simulink model "APP_VD"  (R2016b)
settings: configuration reference "CodeGenConfigSet" (kept outside this file)
values from neighbouring files (symbols this model uses):
  APP_drLinRmp_C = Calibration.Parameter    [init_APP_VD.m]
  APP_facLowNegPT1_C = Calibration.Parameter    [init_APP_VD.m]
  APP_facLowPosPT1_C = Calibration.Parameter    [init_APP_VD.m]
  APP_facMidNegPT1_C = Calibration.Parameter    [init_APP_VD.m]
  APP_facMidPosPT1_C = Calibration.Parameter    [init_APP_VD.m]
  APP_facUppNegPT1_C = Calibration.Parameter    [init_APP_VD.m]
  APP_facUppPosPT1_C = Calibration.Parameter    [init_APP_VD.m]
  APP_rThrFltLowNeg_C = Calibration.Parameter    [init_APP_VD.m]
  APP_rThrFltLowPos_C = Calibration.Parameter    [init_APP_VD.m]
  APP_rThrFltMidNeg_C = Calibration.Parameter    [init_APP_VD.m]
  APP_rThrFltMidPos_C = Calibration.Parameter    [init_APP_VD.m]
  APP_swtEnaFlt_C = Calibration.Parameter    [init_APP_VD.m]
  APP_swtEnaUnJit_C = Calibration.Parameter    [init_APP_VD.m]
  APP_uJitter_C = Calibration.Parameter    [init_APP_VD.m]
  MoFAPP_rLinAPPCURCalMsgA_CUR = Calibration.Parameter    [init_APP_VD.m]
  MoFAPP_rLinAPPCURCalMsgA_CURX = Calibration.Parameter    [init_APP_VD.m]
  SigTst_rAPP_C = Calibration.Parameter    [init_APP_VD.m]
  SigTst_swtAPP_C = Calibration.Parameter    [init_APP_VD.m]
undefined symbols (not defined in the file or in its folder): APP_VD_DT, Switch_conv
libraries: CXLib x4
settings Model: Creator=lenovo  LastModifiedBy=zhoutinglin
settings ConfigSetRef: SourceLocation=Base Workspace

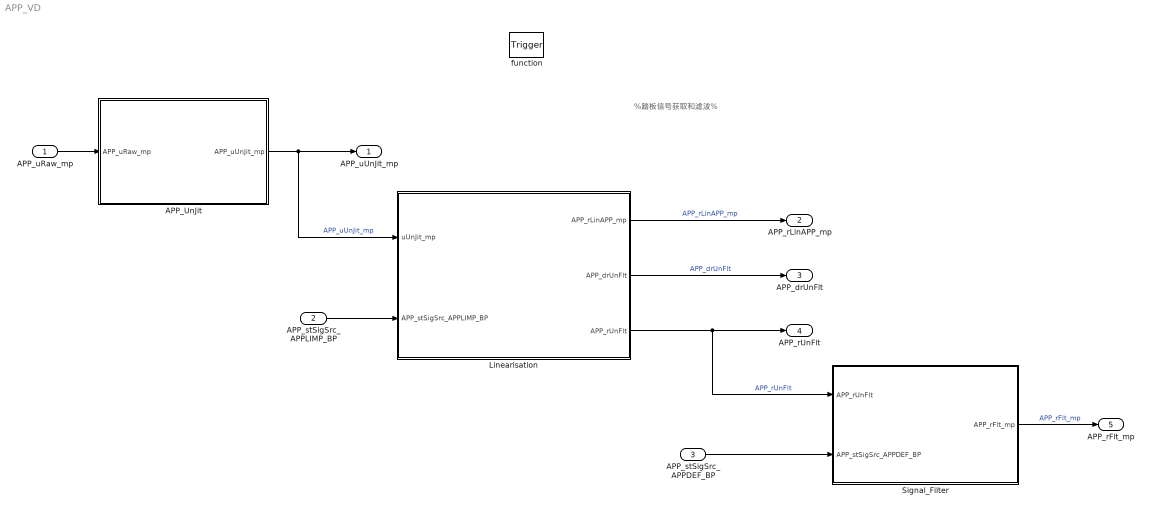
== system APP_VD ==
  note: %踏板信号获取和滤波%
  APP_uRaw_mp : Inport  Tag=mv  Description=Acceleration pedal position raw value  OutMin=0  OutMax=5000  OutDataTypeStr=Ad_mv
  APP_stSigSrc_APPLIMP_BP : Inport  Description=Substitute operation active, accelerator pedal sensor value and accelerator pedal sensor increase are limited  Port=2  OutMin=0  OutMax=1  OutDataTypeStr=boolean
  APP_stSigSrc_APPDEF_BP : Inport  Description=both the sensors are defective. Use the default value  Port=3  OutMin=0  OutMax=1  OutDataTypeStr=boolean
  function : TriggerPort  TriggerType=function-call  VariantControl=Variant
  APP_UnJit : Subsystem
  Linearisation : Subsystem
  Signal_Filter : Subsystem
  APP_uUnJit_mp : Outport  Tag=mv  Description=Acceleration pedal position unjittered value  OutMin=0  OutMax=5000  OutDataTypeStr=Ad_mv
  APP_rLinAPP_mp : Outport  Tag=%  Description=Linearisation ratio of accelerator pedal  Port=2  OutMin=0  OutMax=100  OutDataTypeStr=Accpedal_rate
  APP_drUnFlt : Outport  Tag=%/s  Description=Acceleration pedal position gradient of unfilterd value  Port=3  OutMin=-100000  OutMax=100000  OutDataTypeStr=Accpedal_rate_s
  APP_rUnFlt : Outport  Tag=%  Description=Unfiltered APP value  Port=4  OutMin=0  OutMax=100  OutDataTypeStr=Accpedal_rate
  APP_rFlt_mp : Outport  Tag=%  Description=Acceleration pedal position filtered value  Port=5  OutMin=0  OutMax=100  OutDataTypeStr=Accpedal_rate
  wires:
  APP_uRaw_mp/1 -> APP_UnJit/1(APP_uRaw_mp)
  Linearisation/3(APP_rUnFlt) -> APP_rUnFlt/1, Signal_Filter/1(APP_rUnFlt)  "APP_rUnFlt"
  APP_UnJit/1(APP_uUnJit_mp) -> APP_uUnJit_mp/1, Linearisation/1(uUnJit_mp)  "APP_uUnJit_mp"
  APP_stSigSrc_APPLIMP_BP/1 -> Linearisation/2(APP_stSigSrc_APPLIMP_BP)
  Linearisation/1(APP_rLinAPP_mp) -> APP_rLinAPP_mp/1  "APP_rLinAPP_mp"
  Linearisation/2(APP_drUnFlt) -> APP_drUnFlt/1  "APP_drUnFlt"
  APP_stSigSrc_APPDEF_BP/1 -> Signal_Filter/2(APP_stSigSrc_APPDEF_BP)
  Signal_Filter/1(APP_rFlt_mp) -> APP_rFlt_mp/1  "APP_rFlt_mp"

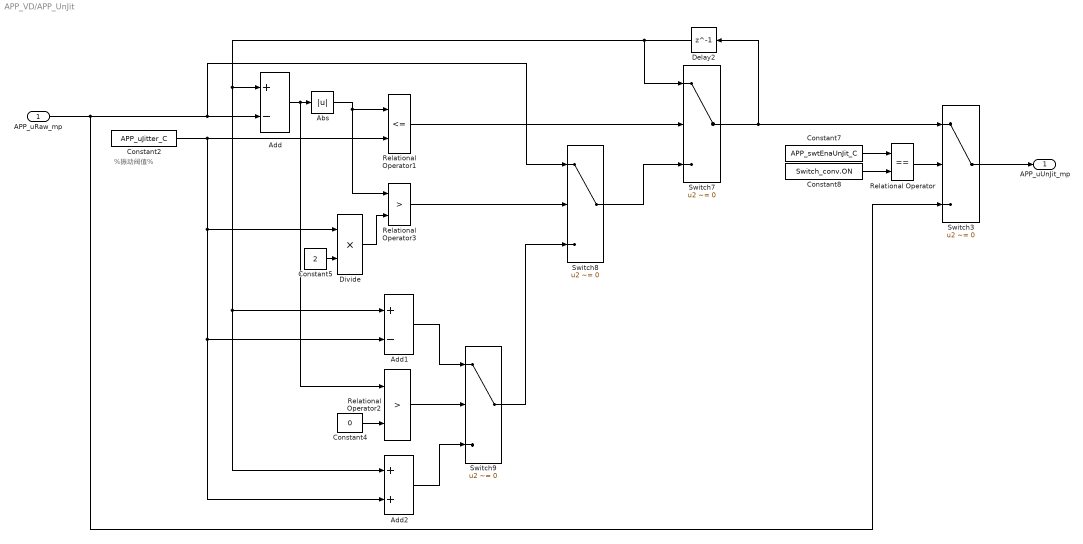
== system APP_VD/APP_UnJit ==
  note: %振动阀值%
  APP_uRaw_mp : Inport
  Abs : Abs  OutDataTypeStr=Inherit: Inherit via back propagation
  Add : Sum  RequirementInfo={'other' 'APP_requirements.doc' '@Simulink_requirement_item_23' 'true' '振动过滤' '' } %GIDa_fc5be5f8_351a_47c4_a4fd_9a4bc0f7c57e  Inputs=+-  InputSameDT=on
  Add1 : Sum  RequirementInfo={'other' 'APP_requirements.doc' '@Simulink_requirement_item_23' 'true' '振动过滤' '' } %GIDa_45ecbb69_9141_4c12_b1d4_2078e7ecff39  Inputs=+-  InputSameDT=on
  Add2 : Sum  RequirementInfo={'other' 'APP_requirements.doc' '@Simulink_requirement_item_23' 'true' '振动过滤' '' } %GIDa_81a4663e_52ce_46e4_8037_be359997c98c  InputSameDT=on
  Constant2 : Constant  RequirementInfo={'other' 'APP_requirements.doc' '@Simulink_requirement_item_23' 'true' '振动过滤' '' } %GIDa_d23093f8_fd9b_402a_9611_6b5f8bec0bd8  Value=APP_uJitter_C
  Constant4 : Constant  Value=0  OutDataTypeStr=Inherit: Inherit via back propagation
  Constant5 : Constant  Value=2  OutDataTypeStr=Inherit: Inherit via back propagation
  Constant7 : Constant  RequirementInfo={'other' 'APP_requirements.doc' '@Simulink_requirement_item_23' 'true' '振动过滤' '' } %GIDa_6fb69985_6827_4f58_8bc8_42b1d63733fd  Value=APP_swtEnaUnJit_C
  Constant8 : Constant  RequirementInfo={'other' 'APP_requirements.doc' '@Simulink_requirement_item_23' 'true' '振动过滤' '' } %GIDa_909ce97d_c784_433c_af86_bcbf068e220e  Value=Switch_conv.ON  OutDataTypeStr=Inherit: Inherit via back propagation
  Delay2 : Delay  RequirementInfo={'other' 'APP_requirements.doc' '@Simulink_requirement_item_23' 'true' '振动过滤' '' } %GIDa_c3bcc4cb_a503_49d7_b00e_b44f6c6fef04  DelayLength=1  InitialCondition=0
  Divide : Product  RequirementInfo={'other' 'APP_requirements.doc' '@Simulink_requirement_item_23' 'true' '振动过滤' '' } %GIDa_c61d8410_39d6_45ff_91b8_1503bdd6ddc8  Inputs=**  OutDataTypeStr=Ad_mv
  Relational Operator : RelationalOperator  Operator===  OutDataTypeStr=boolean  RndMeth=Simplest  InputSameDT=on
  Relational Operator1 : RelationalOperator  RequirementInfo={'other' 'APP_requirements.doc' '@Simulink_requirement_item_23' 'true' '振动过滤' '' } %GIDa_c85495e1_ce88_4564_a155_d6240458c750  Operator=<=  OutDataTypeStr=boolean  RndMeth=Nearest  InputSameDT=on
  Relational Operator2 : RelationalOperator  RequirementInfo={'other' 'APP_requirements.doc' '@Simulink_requirement_item_23' 'true' '振动过滤' '' } %GIDa_dd483711_1e61_4d9e_ab8a_86868d0932d2  Operator=>  OutDataTypeStr=boolean  RndMeth=Nearest  InputSameDT=on
  Relational Operator3 : RelationalOperator  RequirementInfo={'other' 'APP_requirements.doc' '@Simulink_requirement_item_23' 'true' '振动过滤' '' } %GIDa_f6939074_a0b9_4677_988f_218ed7f83d32  Operator=>  OutDataTypeStr=boolean  RndMeth=Nearest  InputSameDT=on
  Switch3 : Switch  RequirementInfo={'other' 'APP_requirements.doc' '@Simulink_requirement_item_23' 'true' '振动过滤' '' } %GIDa_92ed09e8_eaeb_4517_ba56_a552afbd911b  Criteria=u2 ~= 0  InputSameDT=on
  Switch7 : Switch  RequirementInfo={'other' 'APP_requirements.doc' '@Simulink_requirement_item_23' 'true' '振动过滤' '' } %GIDa_8137cdb5_abbd_4efb_b880_66f0d553ed0b  Criteria=u2 ~= 0  InputSameDT=on
  Switch8 : Switch  RequirementInfo={'other' 'APP_requirements.doc' '@Simulink_requirement_item_23' 'true' '振动过滤' '' } %GIDa_1ae86ec7_946c_47f4_81b9_25c1426336ac  Criteria=u2 ~= 0  InputSameDT=on
  Switch9 : Switch  RequirementInfo={'other' 'APP_requirements.doc' '@Simulink_requirement_item_23' 'true' '振动过滤' '' } %GIDa_a2819aca_f461_45d5_9da9_68ba774e98d9  Criteria=u2 ~= 0  InputSameDT=on
  APP_uUnJit_mp : Outport
  wires:
  Constant2/1 -> Add2/2, Add1/2, Divide/1, Relational Operator1/2
  Relational Operator/1 -> Switch3/2
  Add1/1 -> Switch9/1
  Add2/1 -> Switch9/3
  Add/1 -> Abs/1, Relational Operator2/1
  Abs/1 -> Relational Operator1/1, Relational Operator3/1
  Constant8/1 -> Relational Operator/2
  Switch9/1 -> Switch8/3
  Divide/1 -> Relational Operator3/2
  Relational Operator1/1 -> Switch7/2
  Relational Operator3/1 -> Switch8/2
  Delay2/1 -> Add1/1, Add2/1, Add/1, Switch7/1
  Switch7/1 -> Switch3/1, Delay2/1
  Constant5/1 -> Divide/2
  APP_uRaw_mp/1 -> Switch3/3, Add/2, Switch8/1
  Relational Operator2/1 -> Switch9/2
  Constant4/1 -> Relational Operator2/2
  Switch8/1 -> Switch7/3
  Constant7/1 -> Relational Operator/1
  Switch3/1 -> APP_uUnJit_mp/1

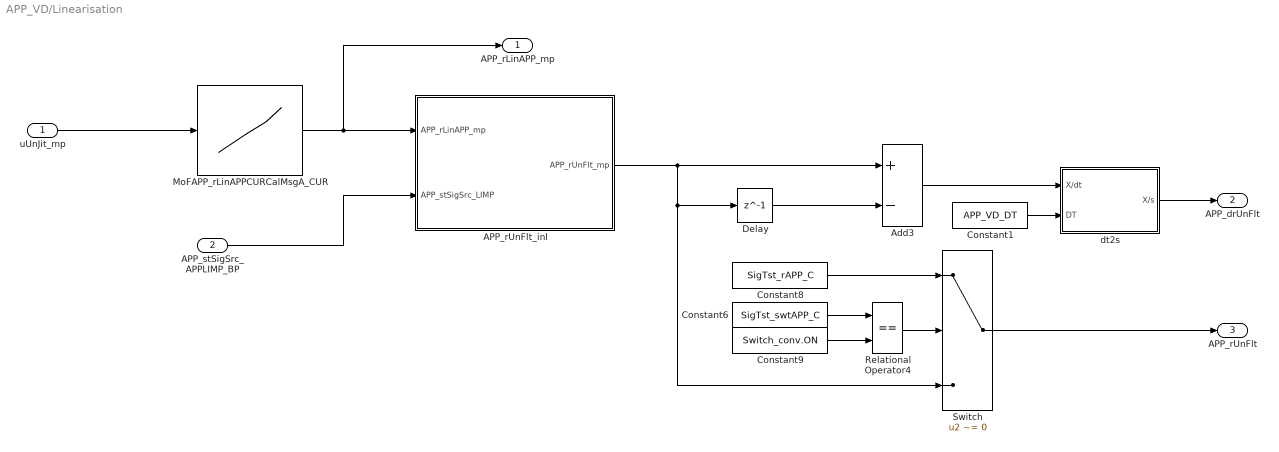
== system APP_VD/Linearisation ==
  uUnJit_mp : Inport
  APP_stSigSrc_APPLIMP_BP : Inport  Tag=-  Description=Substitute operation active, accelerator pedal sensor value and accelerator pedal sensor increase are limited  Port=2  OutMin=0  OutMax=1  OutDataTypeStr=boolean
  APP_rUnFlt_inl : Subsystem
  Add3 : Sum  Inputs=+-  InputSameDT=on
  Constant1 : Constant  RequirementInfo={'other' 'APP_requirements.doc' '@Simulink_requirement_item_25' 'true' '手动开关' '' } %GIDa_76bdba1c_299e_46a3_839d_4b24283771ef  Value=APP_VD_DT  OutDataTypeStr=Inherit: Inherit via back propagation
  Constant6 : Constant  RequirementInfo={'other' 'APP_requirements.doc' '@Simulink_requirement_item_25' 'true' '手动开关' '' } %GIDa_1016d30a_24a7_4f0c_9854_181a7d8dcee6  Value=SigTst_swtAPP_C
  Constant8 : Constant  RequirementInfo={'other' 'APP_requirements.doc' '@Simulink_requirement_item_25' 'true' '手动开关' '' } %GIDa_0d2fb868_9267_4dd8_b106_4322c6fed59f  Value=SigTst_rAPP_C
  Constant9 : Constant  RequirementInfo={'other' 'APP_requirements.doc' '@Simulink_requirement_item_25' 'true' '手动开关' '' } %GIDa_926df48c_1b7c_4174_9563_5ea69c442d0e  Value=Switch_conv.ON  OutDataTypeStr=Inherit: Inherit via back propagation
  Delay : Delay  DelayLength=1  InitialCondition=0
  MoFAPP_rLinAPPCURCalMsgA_CUR : Lookup_n-D  RequirementInfo={'other' 'APP_requirements.doc' '@Simulink_requirement_item_24' 'true' '传感器线性查表' '' } %GIDa_70afb3a8_6904_4b95_98de_7f26b04bbfa0  NumberOfTableDimensions=1  BreakpointsForDimension1=MoFAPP_rLinAPPCURCalMsgA_CURX  IndexSearchMethod=Linear search  BeginIndexSearchUsingPreviousIndexResult=on  UseOneInputPortForAllInputData=on  Table=MoFAPP_rLinAPPCURCalMsgA_CUR  ExtrapMethod=Clip  UseLastTableValue=on  InternalRulePriority=Speed  OutDataTypeStr=Inherit: Inherit via back propagation  SaturateOnIntegerOverflow=on
  Relational Operator4 : RelationalOperator  Operator===  OutDataTypeStr=boolean  RndMeth=Simplest  InputSameDT=on
  Switch : Switch  RequirementInfo={'other' 'APP_requirements.doc' '@Simulink_requirement_item_25' 'true' '手动开关' '' } %GIDa_a1949dba_f114_460f_bb2a_ac25ea53bbd9  Criteria=u2 ~= 0  InputSameDT=on
  dt2s : Subsystem
  APP_rLinAPP_mp : Outport  Tag=%%  Description=Linearisation ratio of accelerator pedal
  APP_drUnFlt : Outport  Tag=%%  Description=Acceleration pedal position gradient of unfilterd value  Port=2
  APP_rUnFlt : Outport  Tag=%%  Description=Unfiltered APP value  Port=3
  wires:
  APP_stSigSrc_APPLIMP_BP/1 -> APP_rUnFlt_inl/2(APP_stSigSrc_LIMP)
  uUnJit_mp/1 -> MoFAPP_rLinAPPCURCalMsgA_CUR/1
  Relational Operator4/1 -> Switch/2
  Constant6/1 -> Relational Operator4/1
  Constant9/1 -> Relational Operator4/2
  Constant8/1 -> Switch/1
  Switch/1 -> APP_rUnFlt/1
  Delay/1 -> Add3/2
  APP_rUnFlt_inl/1(APP_rUnFlt_mp) -> Switch/3, Delay/1, Add3/1
  MoFAPP_rLinAPPCURCalMsgA_CUR/1 -> APP_rLinAPP_mp/1, APP_rUnFlt_inl/1(APP_rLinAPP_mp)
  Constant1/1 -> dt2s/2(DT)
  Add3/1 -> dt2s/1(X/dt)
  dt2s/1(X/s) -> APP_drUnFlt/1

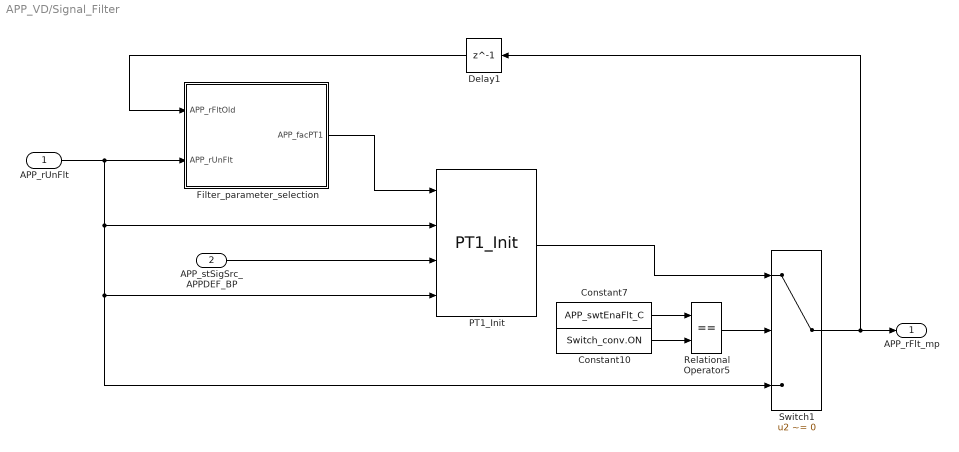
== system APP_VD/Signal_Filter ==
  APP_rUnFlt : Inport
  APP_stSigSrc_APPDEF_BP : Inport  Tag=-  Description=both the sensors are defective. Use the default value  Port=2  OutMin=0  OutMax=1  OutDataTypeStr=boolean
  Constant10 : Constant  RequirementInfo={'other' 'APP_requirements.doc' '@Simulink_requirement_item_25' 'true' '手动开关' '' } %GIDa_63c89112_2158_4769_bece_32f0594febca  Value=Switch_conv.ON  OutDataTypeStr=Inherit: Inherit via back propagation
  Constant7 : Constant  RequirementInfo={'other' 'APP_requirements.doc' '@Simulink_requirement_item_25' 'true' '手动开关' '' } %GIDa_6910ba48_02f2_45bc_af6d_6c6d3576b44f  Value=APP_swtEnaFlt_C
  Delay1 : Delay  DelayLength=1  InitialCondition=0
  Filter_parameter_selection : Subsystem  TreatAsAtomicUnit=on
  PT1_Init : CXLib/PT1_Init  offset=0
  Relational Operator5 : RelationalOperator  Operator===  OutDataTypeStr=boolean  RndMeth=Simplest  InputSameDT=on
  Switch1 : Switch  RequirementInfo={'other' 'APP_requirements.doc' '@Simulink_requirement_item_25' 'true' '手动开关' '' } %GIDa_3d07f01a_8d5a_42a8_96ea_65c61ba5aa22  Criteria=u2 ~= 0  InputSameDT=on
  APP_rFlt_mp : Outport  Tag=%%  Description=Acceleration pedal position filtered value
  wires:
  APP_stSigSrc_APPDEF_BP/1 -> PT1_Init/3
  Relational Operator5/1 -> Switch1/2
  Constant10/1 -> Relational Operator5/2
  Constant7/1 -> Relational Operator5/1
  PT1_Init/1 -> Switch1/1
  Filter_parameter_selection/1(APP_facPT1) -> PT1_Init/1
  Switch1/1 -> APP_rFlt_mp/1, Delay1/1
  Delay1/1 -> Filter_parameter_selection/1(APP_rFltOld)
  APP_rUnFlt/1 -> Switch1/3, PT1_Init/4, PT1_Init/2, Filter_parameter_selection/2(APP_rUnFlt)

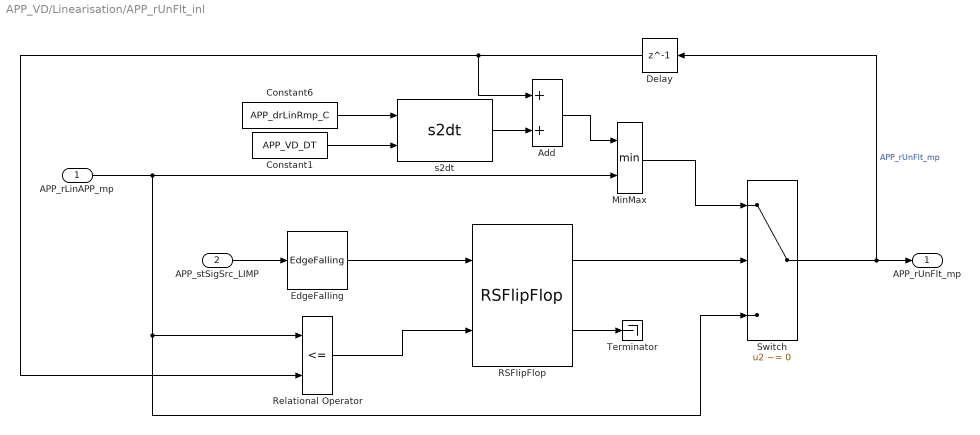
== system APP_VD/Linearisation/APP_rUnFlt_inl ==
  APP_rLinAPP_mp : Inport
  APP_stSigSrc_LIMP : Inport  Port=2
  Add : Sum  InputSameDT=on
  Constant1 : Constant  RequirementInfo={'other' 'APP_requirements.doc' '@Simulink_requirement_item_25' 'true' '手动开关' '' } %GIDa_753f9d75_d861_462f_881b_9418990b68d4  Value=APP_VD_DT  OutDataTypeStr=Inherit: Inherit via back propagation
  Constant6 : Constant  RequirementInfo={'other' 'APP_requirements.doc' '@Simulink_requirement_item_25' 'true' '手动开关' '' } %GIDa_2ce170b2_ab57_4cc2_96f4_304c3052a832  Value=APP_drLinRmp_C
  Delay : Delay  DelayLength=1  InitialCondition=0
  EdgeFalling : CXLib/EdgeFalling
  MinMax : MinMax  Inputs=2
  RSFlipFlop : CXLib/RSFlipFlop
  Relational Operator : RelationalOperator  Operator=<=  OutDataTypeStr=boolean  RndMeth=Simplest
  Switch : Switch  RequirementInfo={'other' 'APP_requirements.doc' '@Simulink_requirement_item_25' 'true' '手动开关' '' } %GIDa_7dc1f05c_2e5d_421b_b7f8_314b6b0d8087  Criteria=u2 ~= 0  InputSameDT=on
  Terminator : Terminator
  s2dt : CXLib/s2dt
  APP_rUnFlt_mp : Outport
  wires:
  RSFlipFlop/2 -> Terminator/1
  Relational Operator/1 -> RSFlipFlop/2
  APP_stSigSrc_LIMP/1 -> EdgeFalling/1
  EdgeFalling/1 -> RSFlipFlop/1
  Delay/1 -> Relational Operator/2, Add/1
  Switch/1 -> APP_rUnFlt_mp/1, Delay/1  "APP_rUnFlt_mp"
  Add/1 -> MinMax/1
  APP_rLinAPP_mp/1 -> MinMax/2, Switch/3, Relational Operator/1
  MinMax/1 -> Switch/1
  RSFlipFlop/1 -> Switch/2
  s2dt/1 -> Add/2
  Constant6/1 -> s2dt/1
  Constant1/1 -> s2dt/2

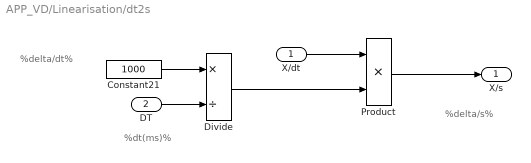
== system APP_VD/Linearisation/dt2s ==
  note: %delta/s%
  note: %delta/dt%
  note: %dt(ms)%
  X/dt : Inport
  DT : Inport  Port=2
  Constant21 : Constant  Value=1000  OutDataTypeStr=int16
  Divide : Product  Inputs=*/  OutDataTypeStr=int16  RndMeth=Round  SaturateOnIntegerOverflow=on
  Product : Product  OutDataTypeStr=Inherit: Inherit via back propagation  RndMeth=Round  SaturateOnIntegerOverflow=on
  X/s : Outport
  wires:
  Product/1 -> X/s/1
  X/dt/1 -> Product/1
  Constant21/1 -> Divide/1
  Divide/1 -> Product/2
  DT/1 -> Divide/2

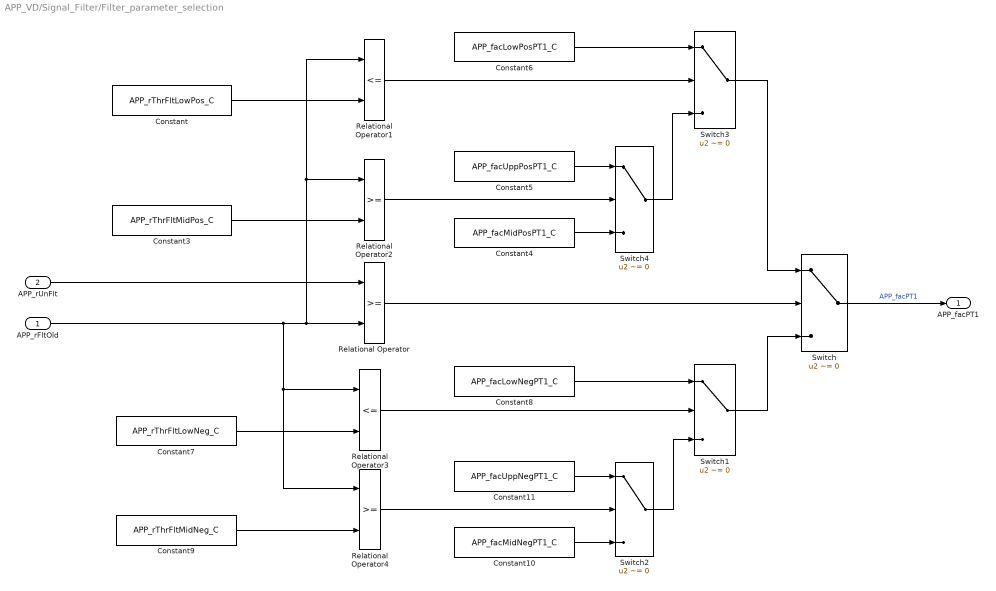
== system APP_VD/Signal_Filter/Filter_parameter_selection ==
  APP_rFltOld : Inport
  APP_rUnFlt : Inport  Port=2
  Constant : Constant  Value=APP_rThrFltLowPos_C
  Constant10 : Constant  Value=APP_facMidNegPT1_C
  Constant11 : Constant  Value=APP_facUppNegPT1_C
  Constant3 : Constant  Value=APP_rThrFltMidPos_C
  Constant4 : Constant  Value=APP_facMidPosPT1_C
  Constant5 : Constant  Value=APP_facUppPosPT1_C
  Constant6 : Constant  Value=APP_facLowPosPT1_C
  Constant7 : Constant  Value=APP_rThrFltLowNeg_C
  Constant8 : Constant  Value=APP_facLowNegPT1_C
  Constant9 : Constant  Value=APP_rThrFltMidNeg_C
  Relational Operator : RelationalOperator  OutDataTypeStr=boolean  RndMeth=Nearest
  Relational Operator1 : RelationalOperator  Operator=<=  OutDataTypeStr=boolean  RndMeth=Nearest
  Relational Operator2 : RelationalOperator  OutDataTypeStr=boolean  RndMeth=Nearest
  Relational Operator3 : RelationalOperator  Operator=<=  OutDataTypeStr=boolean  RndMeth=Nearest
  Relational Operator4 : RelationalOperator  OutDataTypeStr=boolean  RndMeth=Nearest
  Switch{,1..4} (5 alike) : Switch  Criteria=u2 ~= 0  Threshold=1  InputSameDT=on
  APP_facPT1 : Outport
  wires:
  Constant/1 -> Relational Operator1/2
  Constant3/1 -> Relational Operator2/2
  Constant7/1 -> Relational Operator3/2
  Constant9/1 -> Relational Operator4/2
  Relational Operator/1 -> Switch/2
  Constant8/1 -> Switch1/1
  Constant11/1 -> Switch2/1
  Constant10/1 -> Switch2/3
  Relational Operator4/1 -> Switch2/2
  Switch2/1 -> Switch1/3
  Relational Operator3/1 -> Switch1/2
  Constant6/1 -> Switch3/1
  Switch4/1 -> Switch3/3
  Constant5/1 -> Switch4/1
  Constant4/1 -> Switch4/3
  Relational Operator2/1 -> Switch4/2
  Switch3/1 -> Switch/1
  Relational Operator1/1 -> Switch3/2
  APP_rFltOld/1 -> Relational Operator2/1, Relational Operator1/1, Relational Operator/2, Relational Operator3/1, Relational Operator4/1
  APP_rUnFlt/1 -> Relational Operator/1
  Switch1/1 -> Switch/3
  Switch/1 -> APP_facPT1/1  "APP_facPT1"
